simulink model "difference_equation"  (R2020b)
settings: Solver=VariableStepAuto  StartTime=0.0  StopTime=10.0  RelTol=1e-3
settings Model: Creator=shubham sharma  LastModifiedBy=shubham sharma

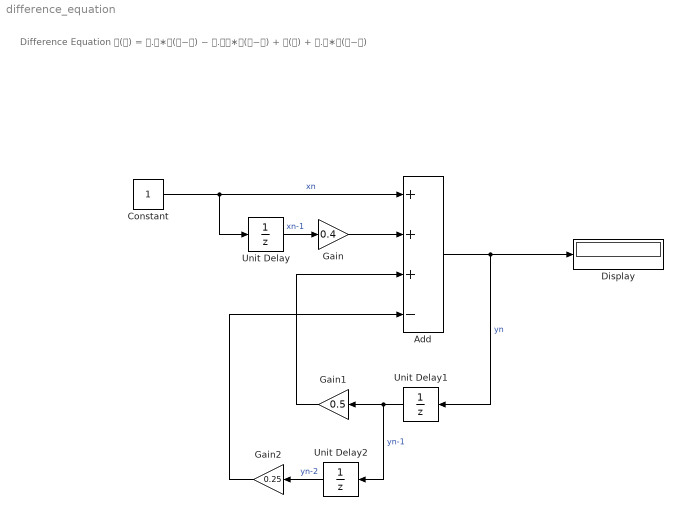
== system difference_equation ==
  note: Difference Equation
      | 𝐲(𝐧) = 𝟎.𝟓∗𝐲(𝐧−𝟏) − 𝟎.𝟐𝟓∗𝐲(𝐧−𝟐) + 𝐱(𝐧) + 𝟎.𝟒∗𝐱(𝐧−𝟏)
  Add : Sum  Inputs=+++-
  Constant : Constant
  Display : Display
  Gain : Gain  Gain=0.4
  Gain1 : Gain  Gain=0.5
  Gain2 : Gain  Gain=0.25
  Unit Delay : UnitDelay  SampleTime=-1  HasFrameUpgradeWarning=on
  Unit Delay1 : UnitDelay  SampleTime=-1  HasFrameUpgradeWarning=on
  Unit Delay2 : UnitDelay  SampleTime=-1  HasFrameUpgradeWarning=on
  wires:
  Constant/1 -> Unit Delay/1, Add/1  "xn"
  Gain/1 -> Add/2
  Unit Delay/1 -> Gain/1  "xn-1"
  Add/1 -> Unit Delay1/1, Display/1  "yn"
  Unit Delay1/1 -> Unit Delay2/1, Gain1/1  "yn-1"
  Gain1/1 -> Add/3
  Unit Delay2/1 -> Gain2/1  "yn-2"
  Gain2/1 -> Add/4
